simulink model "Calculator"  (R2017b)
settings: Solver=FixedStepDiscrete  StartTime=0.0  StopTime=10.0  RelTol=1e-3
settings Model: Creator=Hady Sallam  LastModifiedBy=Hady Sallam
settings OptimizationCC: DefaultParameterBehavior=Inlined  PassReuseOutputArgsAs=Individual arguments
settings DebuggingCC: ParameterTunabilityLossMsg=error
settings SFSimCC: MATLABDynamicMemAlloc=off
settings RTWCC: SystemTargetFile=ert.tlc  GenCodeOnly=on  TemplateMakefile=ert_default_tmf  GenerateReport=on  IncludeHyperlinkInReport=on  LaunchReport=on  GenerateTraceInfo=on  GenerateTraceReport=on  GenerateTraceReportSl=on  GenerateTraceReportSf=on  GenerateTraceReportEml=on
settings CodeAppCC: ForceParamTrailComments=on  IgnoreCustomStorageClasses=off  OperatorAnnotations=on  SimulinkDataObjDesc=on  SFDataObjDesc=on  InsertBlockDesc=on
settings ERTTargetCC: TargetLangStandard=C99 (ISO)  GenerateSampleERTMain=on  InlinedParameterPlacement=NonHierarchical  ERTCustomFileTemplate=example_file_process.tlc  EnableUserReplacementTypes=on

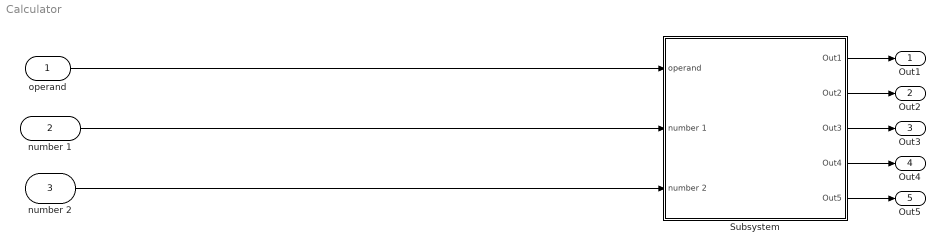
== system Calculator ==
  operand : Inport
  "number 1 " : Inport  Port=2
  number 2 : Inport  Port=3
  Subsystem : Subsystem  TreatAsAtomicUnit=on
      settings: RTWSystemCode=Nonreusable function  RTWFcnNameOpts=Use subsystem name  RTWFileNameOpts=Use subsystem name
  Out1 : Outport
  Out2 : Outport  Port=2
  Out3 : Outport  Port=3
  Out4 : Outport  Port=4
  Out5 : Outport  Port=5
  wires:
  operand/1 -> Subsystem/1(operand)
  "number 1 "/1 -> Subsystem/2("number 1 ")
  number 2/1 -> Subsystem/3(number 2)
  Subsystem/1(Out1) -> Out1/1
  Subsystem/2(Out2) -> Out2/1
  Subsystem/3(Out3) -> Out3/1
  Subsystem/4(Out4) -> Out4/1
  Subsystem/5(Out5) -> Out5/1

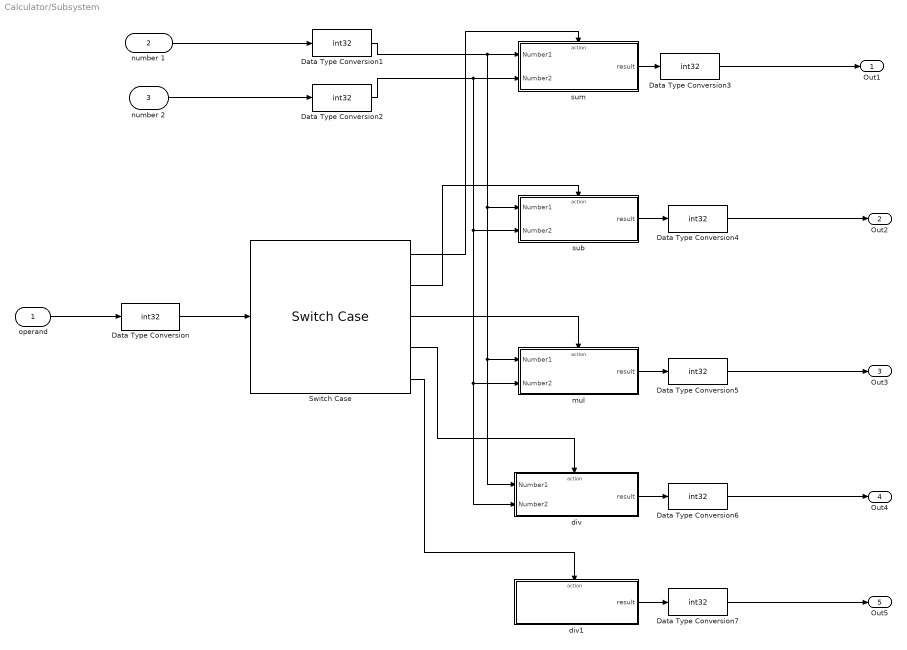
== system Calculator/Subsystem ==
  operand : Inport
  "number 1 " : Inport  Port=2
  number 2 : Inport  Port=3
  Data Type Conversion{,1..7} (8 alike) : DataTypeConversion  OutDataTypeStr=int32
  Switch Case : SwitchCase  CaseConditions={1, 2, 3, 4}
  div : Subsystem  TreatAsAtomicUnit=on
  div1 : Subsystem  TreatAsAtomicUnit=on
  mul : Subsystem  TreatAsAtomicUnit=on
  sub : Subsystem  TreatAsAtomicUnit=on
  sum : Subsystem  TreatAsAtomicUnit=on
  Out1 : Outport
  Out2 : Outport  Port=2
  Out3 : Outport  Port=3
  Out4 : Outport  Port=4
  Out5 : Outport  Port=5
  wires:
  Switch Case/2 -> sub/Action
  "number 1 "/1 -> Data Type Conversion1/1
  div1/1("result ") -> Data Type Conversion7/1
  mul/1("result ") -> Data Type Conversion5/1
  sum/1("result ") -> Data Type Conversion3/1
  Switch Case/1 -> sum/Action
  number 2/1 -> Data Type Conversion2/1
  Data Type Conversion2/1 -> div/2(Number2), mul/2(Number2), sub/2(Number2), sum/2(Number2)
  sub/1(result) -> Data Type Conversion4/1
  Data Type Conversion1/1 -> div/1(Number1), mul/1(Number1), sub/1(Number1), sum/1(Number1)
  div/1("result ") -> Data Type Conversion6/1
  Switch Case/4 -> div/Action
  Switch Case/3 -> mul/Action
  operand/1 -> Data Type Conversion/1
  Data Type Conversion/1 -> Switch Case/1
  Switch Case/5 -> div1/Action
  Data Type Conversion3/1 -> Out1/1
  Data Type Conversion4/1 -> Out2/1
  Data Type Conversion5/1 -> Out3/1
  Data Type Conversion6/1 -> Out4/1
  Data Type Conversion7/1 -> Out5/1

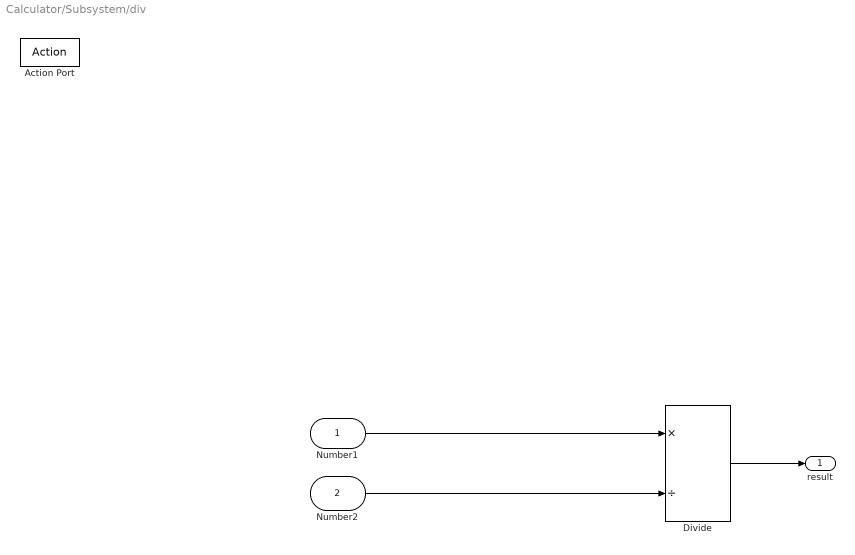
== system Calculator/Subsystem/div ==
  Number1 : Inport
  Number2 : Inport  Port=2
  Action Port : ActionPort  ActionType=case
  Divide : Product  Inputs=*/
  "result " : Outport
  wires:
  Number1/1 -> Divide/1
  Number2/1 -> Divide/2
  Divide/1 -> "result "/1

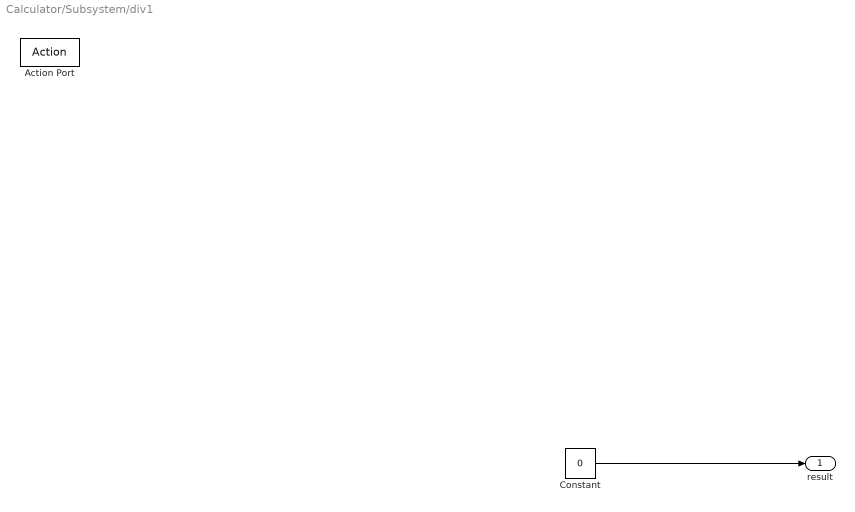
== system Calculator/Subsystem/div1 ==
  Action Port : ActionPort  ActionType=default
  Constant : Constant  Value=0
  "result " : Outport
  wires:
  Constant/1 -> "result "/1

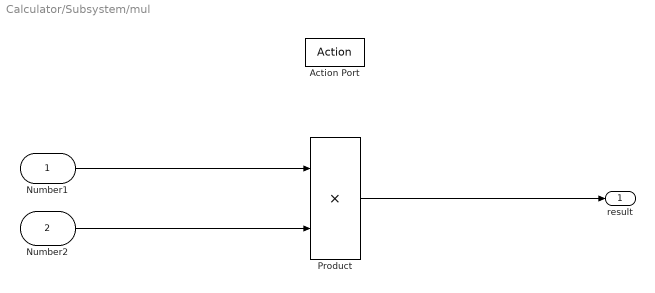
== system Calculator/Subsystem/mul ==
  Number1 : Inport
  Number2 : Inport  Port=2
  Action Port : ActionPort  ActionType=case
  Product : Product
  "result " : Outport
  wires:
  Number1/1 -> Product/1
  Number2/1 -> Product/2
  Product/1 -> "result "/1

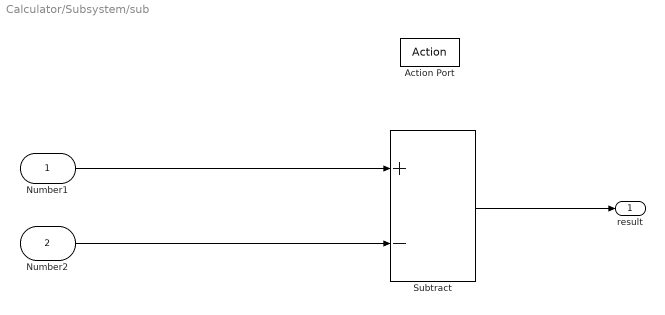
== system Calculator/Subsystem/sub ==
  Number1 : Inport
  Number2 : Inport  Port=2
  Action Port : ActionPort  ActionType=case
  Subtract : Sum  Inputs=+-
  result : Outport
  wires:
  Number1/1 -> Subtract/1
  Number2/1 -> Subtract/2
  Subtract/1 -> result/1

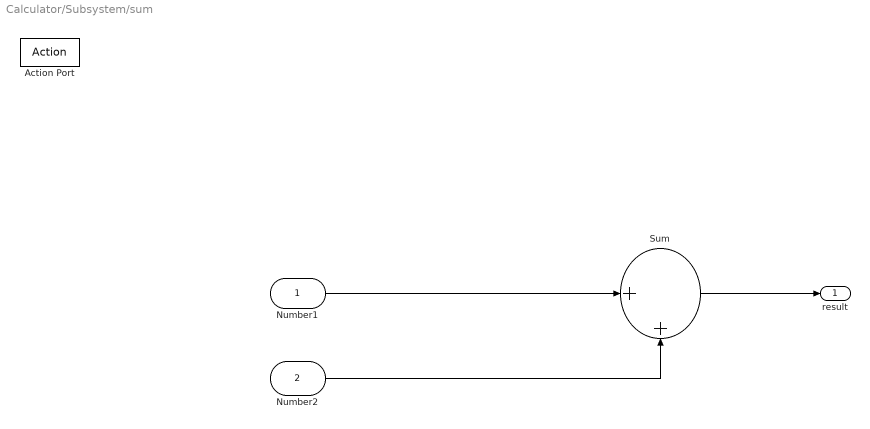
== system Calculator/Subsystem/sum ==
  Number1 : Inport
  Number2 : Inport  Port=2
  Action Port : ActionPort  ActionType=case
  Sum : Sum  Inputs=|++
  "result " : Outport
  wires:
  Sum/1 -> "result "/1
  Number2/1 -> Sum/2
  Number1/1 -> Sum/1
